simulink model "DiscreteSystem"  (R2018b)
settings: Solver=VariableStepAuto  StartTime=0.0  StopTime=500  RelTol=1e-3
settings Model: Creator=soren  LastModifiedBy=soren

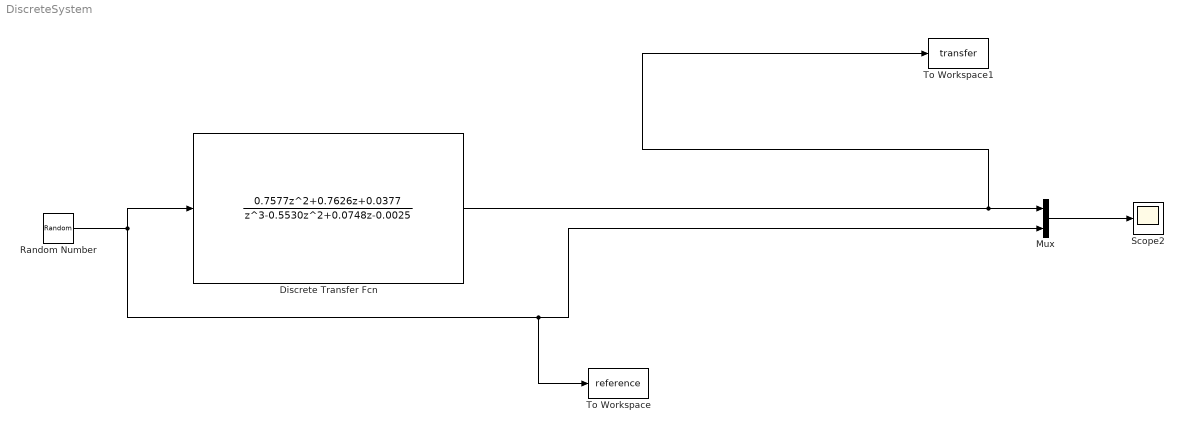
== system DiscreteSystem ==
  Discrete Transfer Fcn : DiscreteTransferFcn  Numerator="[0    0.7577    0.7626    0.0377]"  Denominator="[1.0000   -0.5530    0.0748   -0.0025]"
  Mux : Mux  Inputs=2
  Random Number : RandomNumber  SampleTime=1
  Scope2 : Scope
  To Workspace : ToWorkspace  VariableName=reference  SaveFormat=Timeseries  SampleTime=-1
  To Workspace1 : ToWorkspace  VariableName=transfer  SaveFormat=Timeseries  SampleTime=-1
  wires:
  Discrete Transfer Fcn/1 -> To Workspace1/1, Mux/1
  Random Number/1 -> Discrete Transfer Fcn/1, To Workspace/1, Mux/2
  Mux/1 -> Scope2/1
